simulink model "QiMotorController_ModelReference"  (R2021b)
settings: Solver=FixedStepDiscrete  StartTime=0.0  StopTime=5  RelTol=1e-3
PreLoadFcn:
  | RTWConfigurationCB('preloadfcn', bdroot);
PostLoadFcn:
  | load('configuration/data_struct.mat');
  | load('configuration/fluxMaps_propMotor.mat');
  | load('configuration/parameterInit_PROP.mat');
  | load('configuration/parameterInit_PUMP.mat');
  | load('configuration/parameterInit_PITCH.mat');
  | load('configuration/parameterInit_TILT.mat');
  | %load('configuration/base_workspace_signal_definition.mat');
  | %load('resolvedatastores_to_baseworkspace_for_faster_simulation.mat');
model workspace (MAT data in the model file):
  ADC_CALIBRATION_SAMPLES : Simulink.Parameter (value not decoded)
  DEFAULT_RESOLVER_CONTROL_WORD : Simulink.Parameter (value not decoded)
  PLL_FREQUENCY : Simulink.Parameter (value not decoded)
  SIMULATION_OPTIONS : Simulink.Parameter (value not decoded)
  TARGET_CODE_GEN : Simulink.Parameter (value not decoded)
  Ts = 2.5e-07
symbols that are objects in the model workspace (value not decoded): PLL_FREQUENCY, TARGET_CODE_GEN
undefined symbols (not defined in the file): DEADTIME_NS__PITCH, DEADTIME_NS__PROP, DEADTIME_NS__PUMP, DEADTIME_NS__TILT, fIa_, fIb_, fIc_, fIdc_, fMotorEncoderFloat_, fMotorSensorSpeed_, fUa_, fUb_, fUc_, fUdc_, inbtilt, mdl_pitch_uiAPUFlags, mdl_pitch_uiFlags, modelData, oMot_, oOut_, opInputResolverData_, oPitch, oState_, PLANT_SPEED_QUADRATIC_COEFF__PUMP, POLE_PAIRS_INIT__PITCH, POLE_PAIRS_INIT__PROP, POLE_PAIRS_INIT__PUMP, POLE_PAIRS_INIT__TILT, PWM_FREQ_KHZ__PITCH, PWM_FREQ_KHZ__PROP, PWM_FREQ_KHZ__PUMP, R_PHASE_INIT__PITCH, R_PHASE_INIT__PROP, R_PHASE_INIT__TILT, R_PHASE_INIT_PLANT__PUMP, uiControlReadback_, uiGateDriverStatus_
libraries: simulink x51, spsSeriesRLCBranchLib x25, spsMosfetLib x24, powerlib_extras x24, spsCurrentMeasurementLib x17, spsVoltageMeasurementLib x17, spsPermanentMagnetSynchronousMachineLib x3, spsDCVoltageSourceLib x2, motorModelLibrary x2, slpidlib x2, cstblocks x1, spspowerguiLib x1
(part 5 of 5)

== system QiMotorController_ModelReference/Fault Injection/pitchMotor_faults/Phase Current & Aux Disturbances/Set uiFlags for Aux Trips ==
  note: If an auxiliary trip is to be simulated, set the appropriate uiFlags status.
      | Otherwise, simply pass through the value.
  note: For 1036 fault, uiFlags = 0000 0101
  note: For 1037 fault, uiFlags = 0000 0110 OR 0000 1100
  auxTripCode : Inport
  uiFlags : Inport  Port=2
  Constant : Constant  Value=1036  OutDataTypeStr=uint32  SampleTime=-1
  Constant2 : Constant  Value=5  OutDataTypeStr=uint32  SampleTime=-1
  Constant3 : Constant  Value=1037  OutDataTypeStr=uint32  SampleTime=-1
  Constant4 : Constant  Value=6  OutDataTypeStr=uint32  SampleTime=-1
  Constant5 : Constant  Value=1038  OutDataTypeStr=uint32  SampleTime=-1
  Constant6 : Constant  Value=20  OutDataTypeStr=uint32  SampleTime=-1
  Constant7 : Constant  Value=1039  OutDataTypeStr=uint32  SampleTime=-1
  Constant8 : Constant  Value=7  OutDataTypeStr=uint32  SampleTime=-1
  Equal{,1..3} (4 alike) : RelationalOperator  Operator===  OutDataTypeStr=boolean  RndMeth=Simplest
  Switch{,1,3..4} (4 alike) : Switch  Criteria=u2 > Threshold
  uiFlags_fault : Outport
  wires:
  Constant/1 -> Equal/1
  Equal/1 -> Switch/2
  Constant2/1 -> Switch/1
  Switch/1 -> uiFlags_fault/1
  uiFlags/1 -> Switch4/3
  Constant3/1 -> Equal1/1
  auxTripCode/1 -> Equal/2, Equal1/2, Equal3/2, Equal2/2
  Equal1/1 -> Switch1/2
  Switch1/1 -> Switch/3
  Constant4/1 -> Switch1/1
  Switch3/1 -> Switch1/3
  Constant5/1 -> Equal2/1
  Equal2/1 -> Switch3/2
  Constant6/1 -> Switch3/1
  Constant7/1 -> Equal3/1
  Equal3/1 -> Switch4/2
  Constant8/1 -> Switch4/1
  Switch4/1 -> Switch3/3

== system QiMotorController_ModelReference/Fault Injection/pitchMotor_faults/Phase Current & Aux Disturbances/Set uiGateDriverStatus for Aux Trips ==
  note: If an auxiliary trip is to be simulated, set the appropriate gate driver status (flags).
      | Otherwise, simply pass through the value.
  auxTripCode : Inport
  uiGateDriverStatus : Inport  Port=2
  AND : Logic  AllPortsSameDT=off  OutDataTypeStr=boolean
  Constant1 : Constant  Value=32  OutDataTypeStr=uint32  SampleTime=-1
  Constant10 : Constant  Value=64  OutDataTypeStr=uint32  SampleTime=-1
  Constant11 : Constant  Value=1018  OutDataTypeStr=uint32  SampleTime=-1
  Constant2 : Constant  Value=112  OutDataTypeStr=uint32  SampleTime=-1
  Constant3 : Constant  Value=1036  OutDataTypeStr=uint32  SampleTime=-1
  Constant4 : Constant  Value=1039  OutDataTypeStr=uint32  SampleTime=-1
  Constant5 : Constant  Value=1015  OutDataTypeStr=uint32  SampleTime=-1
  Constant6 : Constant  Value=16  OutDataTypeStr=uint32  SampleTime=-1
  Constant7 : Constant  Value=1017  OutDataTypeStr=uint32  SampleTime=-1
  Constant8 : Constant  Value=1035  OutDataTypeStr=uint32  SampleTime=-1
  Constant9 : Constant  Value=1034  OutDataTypeStr=uint32  SampleTime=-1
  Equal : RelationalOperator  Operator=<=  OutDataTypeStr=boolean  RndMeth=Simplest
  Equal{1..5} (5 alike) : RelationalOperator  Operator===  OutDataTypeStr=boolean  RndMeth=Simplest
  GreaterThanOrEqual : RelationalOperator  OutDataTypeStr=boolean  RndMeth=Simplest
  OR : Logic  Operator=OR  Inputs=3  AllPortsSameDT=off  OutDataTypeStr=boolean
  Switch{1..2,4..5} (4 alike) : Switch  Criteria=u2 > Threshold
  uiGateDriverStatus_fault : Outport
  wires:
  Constant7/1 -> Equal2/2
  Constant9/1 -> Equal4/2
  OR/1 -> Switch5/2
  Constant10/1 -> Switch5/1
  Equal3/1 -> OR/3
  Equal4/1 -> OR/2
  Equal2/1 -> OR/1
  uiGateDriverStatus/1 -> Switch5/3
  Constant8/1 -> Equal3/2
  Switch5/1 -> Switch4/3
  Constant5/1 -> Equal1/2
  Constant6/1 -> Switch4/1
  Equal1/1 -> Switch4/2
  Constant3/1 -> GreaterThanOrEqual/2
  GreaterThanOrEqual/1 -> AND/2
  Constant1/1 -> Switch2/1
  AND/1 -> Switch2/2
  Equal/1 -> AND/1
  Constant4/1 -> Equal/2
  Switch4/1 -> Switch2/3
  Switch2/1 -> Switch1/3
  Constant2/1 -> Switch1/1
  Switch1/1 -> uiGateDriverStatus_fault/1
  Equal5/1 -> Switch1/2
  auxTripCode/1 -> Equal5/1, Equal1/1, Equal3/1, Equal4/1, Equal2/1, GreaterThanOrEqual/1, Equal/1
  Constant11/1 -> Equal5/2

== system QiMotorController_ModelReference/InboardTiltDragLaw2/drag2/load/direct_efficiency ==
  Bus Element In : Inport  PortName=table_efficiency
  Bus Element In1 : Inport  Port=2  PortName=velocity_m
  Bus Element In3 : Inport  Port=2  PortName=velocity_m
  Bus Element In2 : Inport  Port=3  PortName=ideal_load_torque_m
  AND : Logic  IconShape=distinctive  AllPortsSameDT=off  OutDataTypeStr=boolean
  Abs : Abs
  Constant : Constant  Commented=on  Value=10
  Constant1 : Constant  Value=0.45
  Constant3 : Constant  Value=0.05
  Discrete Varying Lowpass : cstblocks/Linear Parameter Varying/Discrete Varying Lowpass  Commented=on  N=1  w0=0  Ts=modelData.Parameters.HighFidelityActuator.SampleTime
      settings: SourceProductBaseCode=CT
  Equal1 : RelationalOperator  Operator===  OutDataTypeStr=boolean  RndMeth=Simplest
  GreaterThan : RelationalOperator  Operator=>  OutDataTypeStr=boolean  RndMeth=Simplest
  Saturation3 : Saturate  UpperLimit=0.99  LowerLimit=0.35
  Saturation4 : Saturate  UpperLimit=0.95  LowerLimit=0.35
  Sign : Signum
  Sign2 : Signum
  Sum : Sum  Inputs=|++
  Sum1 : Sum  Inputs=-+|
  Switch1 : Switch  Criteria=u2 ~= 0
  Zero1 : Constant  Value=1e-1  OutDataTypeStr=Inherit: Inherit via back propagation
  Bus Element Out : Outport  PortName=nominal_efficiency
  wires:
  Switch1/1 -> Bus Element Out/1
  Constant/1 -> Discrete Varying Lowpass/2
  Zero1/1 -> GreaterThan/2
  GreaterThan/1 -> AND/2
  Bus Element In3/1 -> Abs/1
  Abs/1 -> GreaterThan/1
  AND/1 -> Switch1/2  "aiding"
  Constant3/1 -> Sum1/1
  Sum1/1 -> Saturation4/1
  Bus Element In1/1 -> Sign2/1
  Equal1/1 -> AND/1
  Sign/1 -> Equal1/1
  Bus Element In2/1 -> Sign/1
  Saturation3/1 -> Switch1/1  "ehigh"
  Bus Element In/1 -> Sum1/2, Sum/1  "e_table"
  Constant1/1 -> Sum/2
  Sum/1 -> Saturation3/1
  Sign2/1 -> Equal1/2
  Saturation4/1 -> Switch1/3  "elow"

== system QiMotorController_ModelReference/InboardTiltDragLaw2/drag2/load/indirect_efficiency_reduction ==
  Bus Element In2 : Inport  PortName=torque_load_m
  1-D Lookup Table2 : Lookup_n-D  NumberOfTableDimensions=1  BreakpointsForDimension1=(0:100:1000)/161  Table=[1.0, 1.0, 1.0, 0.85, 0.70, 0.50, 0.55, 0.80, 0.90, 0.90, 0.95]  InternalRulePriority=Speed  RndMeth=Simplest  InputSameDT=on
  Abs1 : Abs
  Constant : Constant
  Saturation1 : Saturate  UpperLimit=1  LowerLimit=0.45
  Switch : Switch  Criteria=u2 > Threshold  Threshold=1000/161
  Bus Element Out : Outport  PortName=efficiency_load_reduction
  wires:
  Switch/1 -> Saturation1/1
  1-D Lookup Table2/1 -> Switch/3
  Constant/1 -> Switch/1
  Abs1/1 -> Switch/2, 1-D Lookup Table2/1
  Bus Element In2/1 -> Abs1/1
  Saturation1/1 -> Bus Element Out/1  "em"

== system QiMotorController_ModelReference/Signal Conditioning/qi_dsm_to_sinc1/compute_sinc3_output/Subsystem ==
  In1 : Inport
  l_bits : Inport  Port=2
  decimation_rate : Inport  Port=3
  enable_gain_correction : Inport  Port=4
  Enable : EnablePort
  Add6 : Sum  Inputs=+-
  Add7 : Sum  Inputs=+-
  Add8 : Sum  Inputs=+-
  Constant : Constant  Value=3  OutDataTypeStr=single
  Data Type Conversion2 : DataTypeConversion  OutDataTypeStr=int32
  Data Type Conversion3 : DataTypeConversion  OutDataTypeStr=int32
  Data Type Conversion4 : DataTypeConversion  OutDataTypeStr=int32
  Divide : Product  Inputs=*/
  Power : Math  Operator=pow  SaturateOnIntegerOverflow=on
  Shift Arithmetic : ArithShift  BitShiftNumberSource=Input port  BitShiftNumber=8  BitShiftDirection=Left
      settings: InputPortMap=u0,p1
  Shift Arithmetic1 : ArithShift  BitShiftNumberSource=Input port  BitShiftNumber=8  BitShiftDirection=Right
      settings: InputPortMap=u0,p1
  Switch : Switch  Criteria=u2 > Threshold
  Unit Delay4 : UnitDelay  SampleTime=-1  HasFrameUpgradeWarning=on
  Unit Delay5 : UnitDelay  SampleTime=-1  HasFrameUpgradeWarning=on
  Unit Delay6 : UnitDelay  SampleTime=-1  HasFrameUpgradeWarning=on
  out_sig : Outport
  wires:
  Unit Delay5/1 -> Add7/2
  [comb2] -> Unit Delay6/1
  [comb1] -> Unit Delay5/1
  [comb0] -> Unit Delay4/1
  In1/1 -> [comb0], Add6/1
  Unit Delay6/1 -> Add8/2
  Unit Delay4/1 -> Add6/2
  Add8/1 -> Data Type Conversion2/1
  Add6/1 -> Data Type Conversion3/1
  l_bits/1 -> Shift Arithmetic/2, Shift Arithmetic1/2
  Shift Arithmetic/1 -> Shift Arithmetic1/1
  enable_gain_correction/1 -> Switch/2
  decimation_rate/1 -> Power/1
  Constant/1 -> Power/2
  Power/1 -> Divide/2
  Shift Arithmetic1/1 -> Switch/3, Divide/1
  Divide/1 -> Switch/1
  Data Type Conversion2/1 -> Shift Arithmetic/1, [comb2_out]
  Data Type Conversion4/1 -> [comb2], Add8/1, [comb1_out]
  Add7/1 -> Data Type Conversion4/1
  Data Type Conversion3/1 -> Add7/1, [comb1], [comb0_out]
  Switch/1 -> out_sig/1

== system QiMotorController_ModelReference/Signal Conditioning/qi_dsm_to_sinc1/compute_sinc3_output/log2 ==
  In1 : Inport
  Constant2 : Constant  Value=2  OutDataTypeStr=single
  Divide : Product  Inputs=*/
  Log : Math  Operator=log10  SaturateOnIntegerOverflow=on
  Log1 : Math  Operator=log10  SaturateOnIntegerOverflow=on
  Out1 : Outport
  wires:
  Constant2/1 -> Log/1
  In1/1 -> Log1/1
  Log1/1 -> Divide/1
  Log/1 -> Divide/2
  Divide/1 -> Out1/1

== system QiMotorController_ModelReference/Signal Conditioning/qi_dsm_to_sinc2/compute_sinc3_output/Subsystem ==
  In1 : Inport
  l_bits : Inport  Port=2
  decimation_rate : Inport  Port=3
  enable_gain_correction : Inport  Port=4
  Enable : EnablePort
  Add6 : Sum  Inputs=+-
  Add7 : Sum  Inputs=+-
  Add8 : Sum  Inputs=+-
  Constant : Constant  Value=3  OutDataTypeStr=single
  Data Type Conversion2 : DataTypeConversion  OutDataTypeStr=int32
  Data Type Conversion3 : DataTypeConversion  OutDataTypeStr=int32
  Data Type Conversion4 : DataTypeConversion  OutDataTypeStr=int32
  Divide : Product  Inputs=*/
  Power : Math  Operator=pow  SaturateOnIntegerOverflow=on
  Shift Arithmetic : ArithShift  BitShiftNumberSource=Input port  BitShiftNumber=8  BitShiftDirection=Left
      settings: InputPortMap=u0,p1
  Shift Arithmetic1 : ArithShift  BitShiftNumberSource=Input port  BitShiftNumber=8  BitShiftDirection=Right
      settings: InputPortMap=u0,p1
  Switch : Switch  Criteria=u2 > Threshold
  Unit Delay4 : UnitDelay  SampleTime=-1  HasFrameUpgradeWarning=on
  Unit Delay5 : UnitDelay  SampleTime=-1  HasFrameUpgradeWarning=on
  Unit Delay6 : UnitDelay  SampleTime=-1  HasFrameUpgradeWarning=on
  out_sig : Outport
  wires:
  Unit Delay5/1 -> Add7/2
  [comb2] -> Unit Delay6/1
  [comb1] -> Unit Delay5/1
  [comb0] -> Unit Delay4/1
  In1/1 -> [comb0], Add6/1
  Unit Delay6/1 -> Add8/2
  Unit Delay4/1 -> Add6/2
  Add8/1 -> Data Type Conversion2/1
  Add6/1 -> Data Type Conversion3/1
  l_bits/1 -> Shift Arithmetic/2, Shift Arithmetic1/2
  Shift Arithmetic/1 -> Shift Arithmetic1/1
  enable_gain_correction/1 -> Switch/2
  decimation_rate/1 -> Power/1
  Constant/1 -> Power/2
  Power/1 -> Divide/2
  Shift Arithmetic1/1 -> Switch/3, Divide/1
  Divide/1 -> Switch/1
  Data Type Conversion2/1 -> Shift Arithmetic/1, [comb2_out]
  Data Type Conversion4/1 -> [comb2], Add8/1, [comb1_out]
  Add7/1 -> Data Type Conversion4/1
  Data Type Conversion3/1 -> Add7/1, [comb1], [comb0_out]
  Switch/1 -> out_sig/1

== system QiMotorController_ModelReference/Signal Conditioning/qi_dsm_to_sinc2/compute_sinc3_output/log2 ==
  In1 : Inport
  Constant2 : Constant  Value=2  OutDataTypeStr=single
  Divide : Product  Inputs=*/
  Log : Math  Operator=log10  SaturateOnIntegerOverflow=on
  Log1 : Math  Operator=log10  SaturateOnIntegerOverflow=on
  Out1 : Outport
  wires:
  Constant2/1 -> Log/1
  In1/1 -> Log1/1
  Log1/1 -> Divide/1
  Log/1 -> Divide/2
  Divide/1 -> Out1/1

== system QiMotorController_ModelReference/Signal Conditioning/qi_dsm_to_sinc3/compute_sinc3_output/Subsystem ==
  In1 : Inport
  l_bits : Inport  Port=2
  decimation_rate : Inport  Port=3
  enable_gain_correction : Inport  Port=4
  Enable : EnablePort
  Add6 : Sum  Inputs=+-
  Add7 : Sum  Inputs=+-
  Add8 : Sum  Inputs=+-
  Constant : Constant  Value=3  OutDataTypeStr=single
  Data Type Conversion2 : DataTypeConversion  OutDataTypeStr=int32
  Data Type Conversion3 : DataTypeConversion  OutDataTypeStr=int32
  Data Type Conversion4 : DataTypeConversion  OutDataTypeStr=int32
  Divide : Product  Inputs=*/
  Power : Math  Operator=pow  SaturateOnIntegerOverflow=on
  Shift Arithmetic : ArithShift  BitShiftNumberSource=Input port  BitShiftNumber=8  BitShiftDirection=Left
      settings: InputPortMap=u0,p1
  Shift Arithmetic1 : ArithShift  BitShiftNumberSource=Input port  BitShiftNumber=8  BitShiftDirection=Right
      settings: InputPortMap=u0,p1
  Switch : Switch  Criteria=u2 > Threshold
  Unit Delay4 : UnitDelay  SampleTime=-1  HasFrameUpgradeWarning=on
  Unit Delay5 : UnitDelay  SampleTime=-1  HasFrameUpgradeWarning=on
  Unit Delay6 : UnitDelay  SampleTime=-1  HasFrameUpgradeWarning=on
  out_sig : Outport
  wires:
  Unit Delay5/1 -> Add7/2
  [comb2] -> Unit Delay6/1
  [comb1] -> Unit Delay5/1
  [comb0] -> Unit Delay4/1
  In1/1 -> [comb0], Add6/1
  Unit Delay6/1 -> Add8/2
  Unit Delay4/1 -> Add6/2
  Add8/1 -> Data Type Conversion2/1
  Add6/1 -> Data Type Conversion3/1
  l_bits/1 -> Shift Arithmetic/2, Shift Arithmetic1/2
  Shift Arithmetic/1 -> Shift Arithmetic1/1
  enable_gain_correction/1 -> Switch/2
  decimation_rate/1 -> Power/1
  Constant/1 -> Power/2
  Power/1 -> Divide/2
  Shift Arithmetic1/1 -> Switch/3, Divide/1
  Divide/1 -> Switch/1
  Data Type Conversion2/1 -> Shift Arithmetic/1, [comb2_out]
  Data Type Conversion4/1 -> [comb2], Add8/1, [comb1_out]
  Add7/1 -> Data Type Conversion4/1
  Data Type Conversion3/1 -> Add7/1, [comb1], [comb0_out]
  Switch/1 -> out_sig/1

== system QiMotorController_ModelReference/Signal Conditioning/qi_dsm_to_sinc3/compute_sinc3_output/log2 ==
  In1 : Inport
  Constant2 : Constant  Value=2  OutDataTypeStr=single
  Divide : Product  Inputs=*/
  Log : Math  Operator=log10  SaturateOnIntegerOverflow=on
  Log1 : Math  Operator=log10  SaturateOnIntegerOverflow=on
  Out1 : Outport
  wires:
  Constant2/1 -> Log/1
  In1/1 -> Log1/1
  Log1/1 -> Divide/1
  Log/1 -> Divide/2
  Divide/1 -> Out1/1

== system QiMotorController_ModelReference/Signal Conditioning/qi_dsm_to_sinc4/compute_sinc3_output/Subsystem ==
  In1 : Inport
  l_bits : Inport  Port=2
  decimation_rate : Inport  Port=3
  enable_gain_correction : Inport  Port=4
  Enable : EnablePort
  Add6 : Sum  Inputs=+-
  Add7 : Sum  Inputs=+-
  Add8 : Sum  Inputs=+-
  Constant : Constant  Value=3  OutDataTypeStr=single
  Data Type Conversion2 : DataTypeConversion  OutDataTypeStr=int32
  Data Type Conversion3 : DataTypeConversion  OutDataTypeStr=int32
  Data Type Conversion4 : DataTypeConversion  OutDataTypeStr=int32
  Divide : Product  Inputs=*/
  Power : Math  Operator=pow  SaturateOnIntegerOverflow=on
  Shift Arithmetic : ArithShift  BitShiftNumberSource=Input port  BitShiftNumber=8  BitShiftDirection=Left
      settings: InputPortMap=u0,p1
  Shift Arithmetic1 : ArithShift  BitShiftNumberSource=Input port  BitShiftNumber=8  BitShiftDirection=Right
      settings: InputPortMap=u0,p1
  Switch : Switch  Criteria=u2 > Threshold
  Unit Delay4 : UnitDelay  SampleTime=-1  HasFrameUpgradeWarning=on
  Unit Delay5 : UnitDelay  SampleTime=-1  HasFrameUpgradeWarning=on
  Unit Delay6 : UnitDelay  SampleTime=-1  HasFrameUpgradeWarning=on
  out_sig : Outport
  wires:
  Unit Delay5/1 -> Add7/2
  [comb2] -> Unit Delay6/1
  [comb1] -> Unit Delay5/1
  [comb0] -> Unit Delay4/1
  In1/1 -> [comb0], Add6/1
  Unit Delay6/1 -> Add8/2
  Unit Delay4/1 -> Add6/2
  Add8/1 -> Data Type Conversion2/1
  Add6/1 -> Data Type Conversion3/1
  l_bits/1 -> Shift Arithmetic/2, Shift Arithmetic1/2
  Shift Arithmetic/1 -> Shift Arithmetic1/1
  enable_gain_correction/1 -> Switch/2
  decimation_rate/1 -> Power/1
  Constant/1 -> Power/2
  Power/1 -> Divide/2
  Shift Arithmetic1/1 -> Switch/3, Divide/1
  Divide/1 -> Switch/1
  Data Type Conversion2/1 -> Shift Arithmetic/1, [comb2_out]
  Data Type Conversion4/1 -> [comb2], Add8/1, [comb1_out]
  Add7/1 -> Data Type Conversion4/1
  Data Type Conversion3/1 -> Add7/1, [comb1], [comb0_out]
  Switch/1 -> out_sig/1

== system QiMotorController_ModelReference/Signal Conditioning/qi_dsm_to_sinc4/compute_sinc3_output/log2 ==
  In1 : Inport
  Constant2 : Constant  Value=2  OutDataTypeStr=single
  Divide : Product  Inputs=*/
  Log : Math  Operator=log10  SaturateOnIntegerOverflow=on
  Log1 : Math  Operator=log10  SaturateOnIntegerOverflow=on
  Out1 : Outport
  wires:
  Constant2/1 -> Log/1
  In1/1 -> Log1/1
  Log1/1 -> Divide/1
  Log/1 -> Divide/2
  Divide/1 -> Out1/1

== system QiMotorController_ModelReference/Signal Conditioning/qi_dsm_to_sinc5/compute_sinc3_output/Subsystem ==
  In1 : Inport
  l_bits : Inport  Port=2
  decimation_rate : Inport  Port=3
  enable_gain_correction : Inport  Port=4
  Enable : EnablePort
  Add6 : Sum  Inputs=+-
  Add7 : Sum  Inputs=+-
  Add8 : Sum  Inputs=+-
  Constant : Constant  Value=3  OutDataTypeStr=single
  Data Type Conversion2 : DataTypeConversion  OutDataTypeStr=int32
  Data Type Conversion3 : DataTypeConversion  OutDataTypeStr=int32
  Data Type Conversion4 : DataTypeConversion  OutDataTypeStr=int32
  Divide : Product  Inputs=*/
  Power : Math  Operator=pow  SaturateOnIntegerOverflow=on
  Shift Arithmetic : ArithShift  BitShiftNumberSource=Input port  BitShiftNumber=8  BitShiftDirection=Left
      settings: InputPortMap=u0,p1
  Shift Arithmetic1 : ArithShift  BitShiftNumberSource=Input port  BitShiftNumber=8  BitShiftDirection=Right
      settings: InputPortMap=u0,p1
  Switch : Switch  Criteria=u2 > Threshold
  Unit Delay4 : UnitDelay  SampleTime=-1  HasFrameUpgradeWarning=on
  Unit Delay5 : UnitDelay  SampleTime=-1  HasFrameUpgradeWarning=on
  Unit Delay6 : UnitDelay  SampleTime=-1  HasFrameUpgradeWarning=on
  out_sig : Outport
  wires:
  Unit Delay5/1 -> Add7/2
  [comb2] -> Unit Delay6/1
  [comb1] -> Unit Delay5/1
  [comb0] -> Unit Delay4/1
  In1/1 -> [comb0], Add6/1
  Unit Delay6/1 -> Add8/2
  Unit Delay4/1 -> Add6/2
  Add8/1 -> Data Type Conversion2/1
  Add6/1 -> Data Type Conversion3/1
  l_bits/1 -> Shift Arithmetic/2, Shift Arithmetic1/2
  Shift Arithmetic/1 -> Shift Arithmetic1/1
  enable_gain_correction/1 -> Switch/2
  decimation_rate/1 -> Power/1
  Constant/1 -> Power/2
  Power/1 -> Divide/2
  Shift Arithmetic1/1 -> Switch/3, Divide/1
  Divide/1 -> Switch/1
  Data Type Conversion2/1 -> Shift Arithmetic/1, [comb2_out]
  Data Type Conversion4/1 -> [comb2], Add8/1, [comb1_out]
  Add7/1 -> Data Type Conversion4/1
  Data Type Conversion3/1 -> Add7/1, [comb1], [comb0_out]
  Switch/1 -> out_sig/1

== system QiMotorController_ModelReference/Signal Conditioning/qi_dsm_to_sinc5/compute_sinc3_output/log2 ==
  In1 : Inport
  Constant2 : Constant  Value=2  OutDataTypeStr=single
  Divide : Product  Inputs=*/
  Log : Math  Operator=log10  SaturateOnIntegerOverflow=on
  Log1 : Math  Operator=log10  SaturateOnIntegerOverflow=on
  Out1 : Outport
  wires:
  Constant2/1 -> Log/1
  In1/1 -> Log1/1
  Log1/1 -> Divide/1
  Log/1 -> Divide/2
  Divide/1 -> Out1/1

== system QiMotorController_ModelReference/Signal Conditioning/qi_dsm_to_sinc6/compute_sinc3_output/Subsystem ==
  In1 : Inport
  l_bits : Inport  Port=2
  decimation_rate : Inport  Port=3
  enable_gain_correction : Inport  Port=4
  Enable : EnablePort
  Add6 : Sum  Inputs=+-
  Add7 : Sum  Inputs=+-
  Add8 : Sum  Inputs=+-
  Constant : Constant  Value=3  OutDataTypeStr=single
  Data Type Conversion2 : DataTypeConversion  OutDataTypeStr=int32
  Data Type Conversion3 : DataTypeConversion  OutDataTypeStr=int32
  Data Type Conversion4 : DataTypeConversion  OutDataTypeStr=int32
  Divide : Product  Inputs=*/
  Power : Math  Operator=pow  SaturateOnIntegerOverflow=on
  Shift Arithmetic : ArithShift  BitShiftNumberSource=Input port  BitShiftNumber=8  BitShiftDirection=Left
      settings: InputPortMap=u0,p1
  Shift Arithmetic1 : ArithShift  BitShiftNumberSource=Input port  BitShiftNumber=8  BitShiftDirection=Right
      settings: InputPortMap=u0,p1
  Switch : Switch  Criteria=u2 > Threshold
  Unit Delay4 : UnitDelay  SampleTime=-1  HasFrameUpgradeWarning=on
  Unit Delay5 : UnitDelay  SampleTime=-1  HasFrameUpgradeWarning=on
  Unit Delay6 : UnitDelay  SampleTime=-1  HasFrameUpgradeWarning=on
  out_sig : Outport
  wires:
  Unit Delay5/1 -> Add7/2
  [comb2] -> Unit Delay6/1
  [comb1] -> Unit Delay5/1
  [comb0] -> Unit Delay4/1
  In1/1 -> [comb0], Add6/1
  Unit Delay6/1 -> Add8/2
  Unit Delay4/1 -> Add6/2
  Add8/1 -> Data Type Conversion2/1
  Add6/1 -> Data Type Conversion3/1
  l_bits/1 -> Shift Arithmetic/2, Shift Arithmetic1/2
  Shift Arithmetic/1 -> Shift Arithmetic1/1
  enable_gain_correction/1 -> Switch/2
  decimation_rate/1 -> Power/1
  Constant/1 -> Power/2
  Power/1 -> Divide/2
  Shift Arithmetic1/1 -> Switch/3, Divide/1
  Divide/1 -> Switch/1
  Data Type Conversion2/1 -> Shift Arithmetic/1, [comb2_out]
  Data Type Conversion4/1 -> [comb2], Add8/1, [comb1_out]
  Add7/1 -> Data Type Conversion4/1
  Data Type Conversion3/1 -> Add7/1, [comb1], [comb0_out]
  Switch/1 -> out_sig/1

== system QiMotorController_ModelReference/Signal Conditioning/qi_dsm_to_sinc6/compute_sinc3_output/log2 ==
  In1 : Inport
  Constant2 : Constant  Value=2  OutDataTypeStr=single
  Divide : Product  Inputs=*/
  Log : Math  Operator=log10  SaturateOnIntegerOverflow=on
  Log1 : Math  Operator=log10  SaturateOnIntegerOverflow=on
  Out1 : Outport
  wires:
  Constant2/1 -> Log/1
  In1/1 -> Log1/1
  Log1/1 -> Divide/1
  Log/1 -> Divide/2
  Divide/1 -> Out1/1

== system QiMotorController_ModelReference/Signal Conditioning/qi_dsm_to_sinc7/compute_sinc3_output/Subsystem ==
  In1 : Inport
  l_bits : Inport  Port=2
  decimation_rate : Inport  Port=3
  enable_gain_correction : Inport  Port=4
  Enable : EnablePort
  Add6 : Sum  Inputs=+-
  Add7 : Sum  Inputs=+-
  Add8 : Sum  Inputs=+-
  Constant : Constant  Value=3  OutDataTypeStr=single
  Data Type Conversion2 : DataTypeConversion  OutDataTypeStr=int32
  Data Type Conversion3 : DataTypeConversion  OutDataTypeStr=int32
  Data Type Conversion4 : DataTypeConversion  OutDataTypeStr=int32
  Divide : Product  Inputs=*/
  Power : Math  Operator=pow  SaturateOnIntegerOverflow=on
  Shift Arithmetic : ArithShift  BitShiftNumberSource=Input port  BitShiftNumber=8  BitShiftDirection=Left
      settings: InputPortMap=u0,p1
  Shift Arithmetic1 : ArithShift  BitShiftNumberSource=Input port  BitShiftNumber=8  BitShiftDirection=Right
      settings: InputPortMap=u0,p1
  Switch : Switch  Criteria=u2 > Threshold
  Unit Delay4 : UnitDelay  SampleTime=-1  HasFrameUpgradeWarning=on
  Unit Delay5 : UnitDelay  SampleTime=-1  HasFrameUpgradeWarning=on
  Unit Delay6 : UnitDelay  SampleTime=-1  HasFrameUpgradeWarning=on
  out_sig : Outport
  wires:
  Unit Delay5/1 -> Add7/2
  [comb2] -> Unit Delay6/1
  [comb1] -> Unit Delay5/1
  [comb0] -> Unit Delay4/1
  In1/1 -> [comb0], Add6/1
  Unit Delay6/1 -> Add8/2
  Unit Delay4/1 -> Add6/2
  Add8/1 -> Data Type Conversion2/1
  Add6/1 -> Data Type Conversion3/1
  l_bits/1 -> Shift Arithmetic/2, Shift Arithmetic1/2
  Shift Arithmetic/1 -> Shift Arithmetic1/1
  enable_gain_correction/1 -> Switch/2
  decimation_rate/1 -> Power/1
  Constant/1 -> Power/2
  Power/1 -> Divide/2
  Shift Arithmetic1/1 -> Switch/3, Divide/1
  Divide/1 -> Switch/1
  Data Type Conversion2/1 -> Shift Arithmetic/1, [comb2_out]
  Data Type Conversion4/1 -> [comb2], Add8/1, [comb1_out]
  Add7/1 -> Data Type Conversion4/1
  Data Type Conversion3/1 -> Add7/1, [comb1], [comb0_out]
  Switch/1 -> out_sig/1

== system QiMotorController_ModelReference/Signal Conditioning/qi_dsm_to_sinc7/compute_sinc3_output/log2 ==
  In1 : Inport
  Constant2 : Constant  Value=2  OutDataTypeStr=single
  Divide : Product  Inputs=*/
  Log : Math  Operator=log10  SaturateOnIntegerOverflow=on
  Log1 : Math  Operator=log10  SaturateOnIntegerOverflow=on
  Out1 : Outport
  wires:
  Constant2/1 -> Log/1
  In1/1 -> Log1/1
  Log1/1 -> Divide/1
  Log/1 -> Divide/2
  Divide/1 -> Out1/1

== system QiMotorController_ModelReference/Signal Conditioning/qi_dsm_to_sinc8/compute_sinc3_output/Subsystem ==
  In1 : Inport
  l_bits : Inport  Port=2
  decimation_rate : Inport  Port=3
  enable_gain_correction : Inport  Port=4
  Enable : EnablePort
  Add6 : Sum  Inputs=+-
  Add7 : Sum  Inputs=+-
  Add8 : Sum  Inputs=+-
  Constant : Constant  Value=3  OutDataTypeStr=single
  Data Type Conversion2 : DataTypeConversion  OutDataTypeStr=int32
  Data Type Conversion3 : DataTypeConversion  OutDataTypeStr=int32
  Data Type Conversion4 : DataTypeConversion  OutDataTypeStr=int32
  Divide : Product  Inputs=*/
  Power : Math  Operator=pow  SaturateOnIntegerOverflow=on
  Shift Arithmetic : ArithShift  BitShiftNumberSource=Input port  BitShiftNumber=8  BitShiftDirection=Left
      settings: InputPortMap=u0,p1
  Shift Arithmetic1 : ArithShift  BitShiftNumberSource=Input port  BitShiftNumber=8  BitShiftDirection=Right
      settings: InputPortMap=u0,p1
  Switch : Switch  Criteria=u2 > Threshold
  Unit Delay4 : UnitDelay  SampleTime=-1  HasFrameUpgradeWarning=on
  Unit Delay5 : UnitDelay  SampleTime=-1  HasFrameUpgradeWarning=on
  Unit Delay6 : UnitDelay  SampleTime=-1  HasFrameUpgradeWarning=on
  out_sig : Outport
  wires:
  Unit Delay5/1 -> Add7/2
  [comb2] -> Unit Delay6/1
  [comb1] -> Unit Delay5/1
  [comb0] -> Unit Delay4/1
  In1/1 -> [comb0], Add6/1
  Unit Delay6/1 -> Add8/2
  Unit Delay4/1 -> Add6/2
  Add8/1 -> Data Type Conversion2/1
  Add6/1 -> Data Type Conversion3/1
  l_bits/1 -> Shift Arithmetic/2, Shift Arithmetic1/2
  Shift Arithmetic/1 -> Shift Arithmetic1/1
  enable_gain_correction/1 -> Switch/2
  decimation_rate/1 -> Power/1
  Constant/1 -> Power/2
  Power/1 -> Divide/2
  Shift Arithmetic1/1 -> Switch/3, Divide/1
  Divide/1 -> Switch/1
  Data Type Conversion2/1 -> Shift Arithmetic/1, [comb2_out]
  Data Type Conversion4/1 -> [comb2], Add8/1, [comb1_out]
  Add7/1 -> Data Type Conversion4/1
  Data Type Conversion3/1 -> Add7/1, [comb1], [comb0_out]
  Switch/1 -> out_sig/1

== system QiMotorController_ModelReference/Signal Conditioning/qi_dsm_to_sinc8/compute_sinc3_output/log2 ==
  In1 : Inport
  Constant2 : Constant  Value=2  OutDataTypeStr=single
  Divide : Product  Inputs=*/
  Log : Math  Operator=log10  SaturateOnIntegerOverflow=on
  Log1 : Math  Operator=log10  SaturateOnIntegerOverflow=on
  Out1 : Outport
  wires:
  Constant2/1 -> Log/1
  In1/1 -> Log1/1
  Log1/1 -> Divide/1
  Log/1 -> Divide/2
  Divide/1 -> Out1/1

== matlab function QiMotorController_ModelReference/InboardTiltDragLaw2/Subsystem1/MATLAB Function ==
  data: DrgMlt input; Eta output; n_inv input
function Eta = fcn(DrgMlt, n_inv)
%
%   /// \breif Check in what drag mode we are currently running; this is for tilts only
%   /// Logic table: -1, not floppy; -1 floppy;  use dMechanicalEfficiency_ in the 1st case; in the 2nd, does not matter FD does the calcs
%   ///               0, not floppy;  0 floppy;  use dMechanicalEfficiency_ only for the 1st of the two
%   ///               >0, not floppy; >0 floppy;  do not use dMechanicaEfficiency_ in either mode, i.e. set it to 1Type your documentation here
%   
   
Eta = -1;

% Default simple eta for load transfer to input
if( DrgMlt == -1 && n_inv > 0 )
    Eta = 0.7;
end

% Default simple eta for load transfer to input
if( DrgMlt == 0 && n_inv > 0 )
    Eta = 0.7;
end

% Full drag law. Leave load umodified at input
if ( DrgMlt > 0 && n_inv > 0 )
    Eta = 1;
end

% 'Floppy' tilt condition via unpowered motor; Leave load
% unmodified at input
if( n_inv == 0 )
    Eta = 1;
end

end
